simulink model "P2_Modelo_4_1_MotorIdeal"  (R2023a)
settings: Solver=VariableStepAuto  StartTime=0.0  StopTime=10.0  RelTol=1e-3
undefined symbols (not defined in the file): k_e, p
settings Model: Creator=sisdin  LastModifiedBy=sisdin

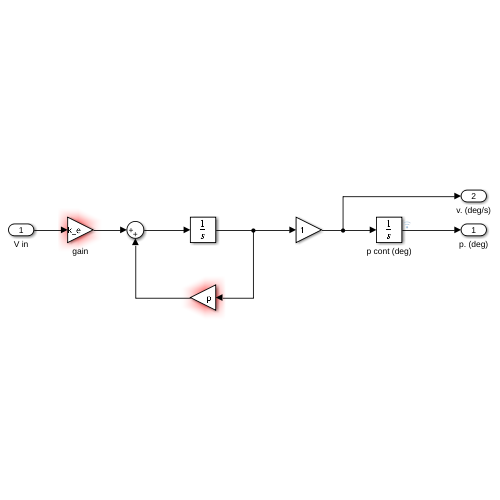
[thumbnail: Simulink's stored preview of the top-level diagram]
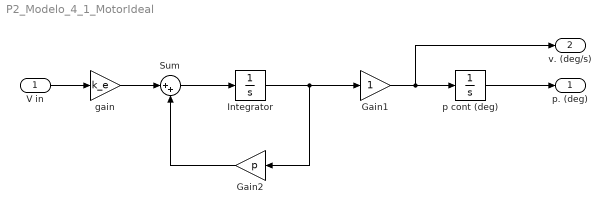
== system P2_Modelo_4_1_MotorIdeal ==
  V in : Inport
  Gain1 : Gain
  Gain2 : Gain  Gain=p
  Integrator : Integrator
  Sum : Sum  Inputs=|++
  gain : Gain  Gain=k_e
  p cont (deg) : Integrator
  p. (deg) : Outport
  v. (deg/s) : Outport  Port=2
  wires:
  V in/1 -> gain/1
  gain/1 -> Sum/1
  Sum/1 -> Integrator/1
  Integrator/1 -> Gain2/1, Gain1/1
  Gain1/1 -> v. (deg/s)/1, p cont (deg)/1
  Gain2/1 -> Sum/2
  p cont (deg)/1 -> p. (deg)/1
